simulink model "Arranque_exp"  (R2018b)
settings: Solver=VariableStepAuto  StartTime=0.0  StopTime=20  MaxStep=1e-4  RelTol=1e-3
values from neighbouring files (symbols this model uses):
  ia = a(:,2)-mean(a(:,2))    [carga_exp.m]
  ia1 = b(:,2)-mean(b(:,2))    [carga_exp.m]
  ib = a(:,4)-mean(a(:,4))    [carga_exp.m]
  ib1 = b(:,4)-mean(b(:,4))    [carga_exp.m]
  ic = a(:,3)-mean(a(:,3))    [carga_exp.m]
  ic1 = b(:,3)-mean(b(:,3))    [carga_exp.m]
  t1 = b(:,1)    [carga_exp.m]
  va = a(:,5)-mean(a(:,5))    [carga_exp.m]
  va1 = b(:,5)-mean(b(:,5))    [carga_exp.m]
  vb = a(:,7)-mean(a(:,7))    [carga_exp.m]
  vb1 = b(:,7)-mean(b(:,7))    [carga_exp.m]
  vc = a(:,6)-mean(a(:,6))    [carga_exp.m]
  vc1 = b(:,6)-mean(b(:,6))    [carga_exp.m]
libraries: powerlib_meascontrol x8
settings Model: Creator=Guille2  LastModifiedBy=grbos
settings SFSimCC: SimUseLocalCustomCode=off
settings RTWCC: RTWUseLocalCustomCode=off

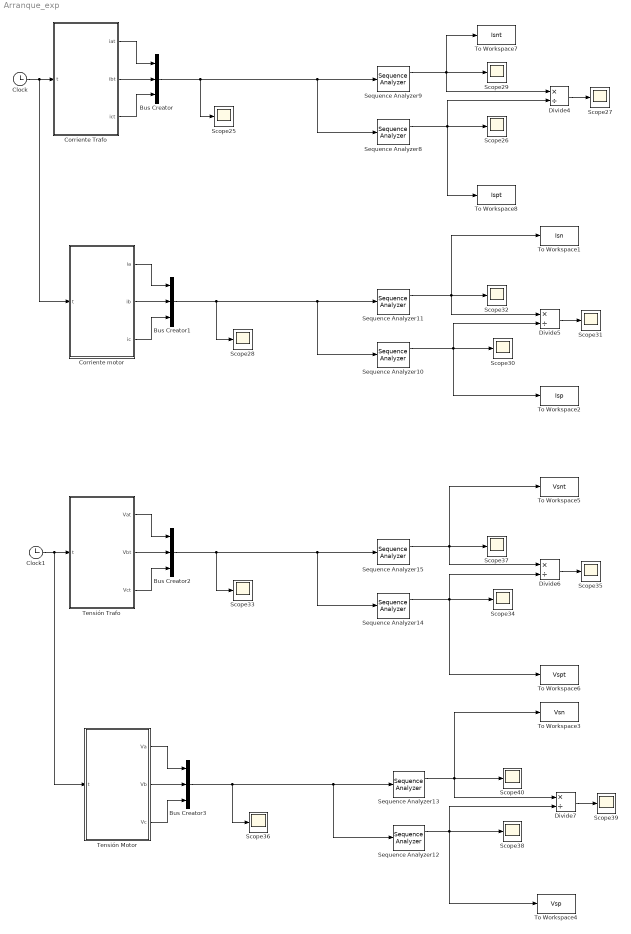
== system Arranque_exp ==
  Bus Creator{,1..3} (4 alike) : BusCreator  Inputs=3
  Clock : Clock
      settings: Decimation=20
  Clock1 : Clock
      settings: Decimation=20
  Corriente Trafo : Subsystem
  Corriente motor : Subsystem
  Divide{4..7} (4 alike) : Product  Inputs=*/
  Scope{25..40} (16 alike) : Scope
  Sequence Analyzer{8,10,12,14} (4 alike) : powerlib_meascontrol/Measurements/Sequence Analyzer  Freq=50  n=1  seq=Positive  InInit=[1, 0]  Ts=0
      settings: SourceProductName=Simscape Electrical  SourceProductBaseCode=PS
  Sequence Analyzer{9,11,13,15} (4 alike) : powerlib_meascontrol/Measurements/Sequence Analyzer  Freq=50  n=1  seq=Negative  InInit=[1, 0]  Ts=0
      settings: SourceProductName=Simscape Electrical  SourceProductBaseCode=PS
  Tensión Motor : Subsystem
  Tensión Trafo : Subsystem
  To Workspace1 : ToWorkspace  VariableName=Isn  SaveFormat=Timeseries  SampleTime=0.001
  To Workspace2 : ToWorkspace  VariableName=Isp  SaveFormat=Timeseries  SampleTime=0.001
  To Workspace3 : ToWorkspace  VariableName=Vsn  SaveFormat=Timeseries  SampleTime=0.001
  To Workspace4 : ToWorkspace  VariableName=Vsp  SaveFormat=Timeseries  SampleTime=0.001
  To Workspace5 : ToWorkspace  VariableName=Vsnt  SaveFormat=Timeseries  SampleTime=0.001
  To Workspace6 : ToWorkspace  VariableName=Vspt  SaveFormat=Timeseries  SampleTime=0.001
  To Workspace7 : ToWorkspace  VariableName=Isnt  SaveFormat=Timeseries  SampleTime=0.001
  To Workspace8 : ToWorkspace  VariableName=Ispt  SaveFormat=Timeseries  SampleTime=0.001
  wires:
  Corriente Trafo/1(iat) -> Bus Creator/1
  Corriente Trafo/2(ibt) -> Bus Creator/2
  Corriente Trafo/3(ict) -> Bus Creator/3
  Bus Creator/1 -> Sequence Analyzer8/1, Sequence Analyzer9/1, Scope25/1
  Clock/1 -> Corriente motor/1(t), Corriente Trafo/1(t)
  Sequence Analyzer8/1 -> Divide4/2, Scope26/1, To Workspace8/1
  Sequence Analyzer9/1 -> Divide4/1, Scope29/1, To Workspace7/1
  Divide4/1 -> Scope27/1
  Divide5/1 -> Scope31/1
  Sequence Analyzer11/1 -> Divide5/1, Scope32/1, To Workspace1/1
  Sequence Analyzer10/1 -> Divide5/2, Scope30/1, To Workspace2/1
  Bus Creator1/1 -> Sequence Analyzer10/1, Sequence Analyzer11/1, Scope28/1
  Corriente motor/1(ia) -> Bus Creator1/1
  Corriente motor/2(ib) -> Bus Creator1/2
  Corriente motor/3(ic) -> Bus Creator1/3
  Clock1/1 -> Tensión Motor/1(t), Tensión Trafo/1(t)
  Tensión Motor/2(Vb) -> Bus Creator3/2
  Tensión Trafo/3(Vct) -> Bus Creator2/3
  Divide6/1 -> Scope35/1
  Divide7/1 -> Scope39/1
  Bus Creator3/1 -> Sequence Analyzer12/1, Sequence Analyzer13/1, Scope36/1
  Tensión Trafo/2(Vbt) -> Bus Creator2/2
  Sequence Analyzer13/1 -> Divide7/1, Scope40/1, To Workspace3/1
  Tensión Trafo/1(Vat) -> Bus Creator2/1
  Sequence Analyzer12/1 -> Divide7/2, Scope38/1, To Workspace4/1
  Sequence Analyzer14/1 -> To Workspace6/1, Divide6/2, Scope34/1
  Tensión Motor/1(Va) -> Bus Creator3/1
  Bus Creator2/1 -> Sequence Analyzer14/1, Sequence Analyzer15/1, Scope33/1
  Tensión Motor/3(Vc) -> Bus Creator3/3
  Sequence Analyzer15/1 -> Divide6/1, Scope37/1, To Workspace5/1

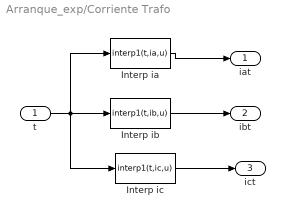
== system Arranque_exp/Corriente Trafo ==
  t : Inport
  Interp ia : MATLABFcn  MATLABFcn=interp1(t,ia,u)  OutputDimensions=1  OutputSignalType=real  Output1D=off
  Interp ib : MATLABFcn  MATLABFcn=interp1(t,ib,u)  OutputDimensions=1  OutputSignalType=real  Output1D=off
  Interp ic : MATLABFcn  MATLABFcn=interp1(t,ic,u)  OutputDimensions=1  Output1D=off
  iat : Outport
  ibt : Outport  Port=2
  ict : Outport  Port=3
  wires:
  Interp ia/1 -> iat/1
  Interp ib/1 -> ibt/1
  t/1 -> Interp ia/1, Interp ib/1, Interp ic/1
  Interp ic/1 -> ict/1

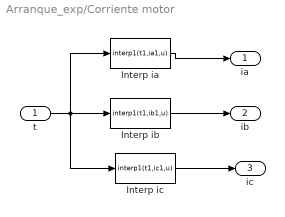
== system Arranque_exp/Corriente motor ==
  t : Inport
  Interp ia : MATLABFcn  MATLABFcn=interp1(t1,ia1,u)  OutputDimensions=1  OutputSignalType=real  Output1D=off
  Interp ib : MATLABFcn  MATLABFcn=interp1(t1,ib1,u)  OutputDimensions=1  OutputSignalType=real  Output1D=off
  Interp ic : MATLABFcn  MATLABFcn=interp1(t1,ic1,u)  OutputDimensions=1  Output1D=off
  ia : Outport
  ib : Outport  Port=2
  ic : Outport  Port=3
  wires:
  Interp ia/1 -> ia/1
  Interp ib/1 -> ib/1
  t/1 -> Interp ia/1, Interp ib/1, Interp ic/1
  Interp ic/1 -> ic/1

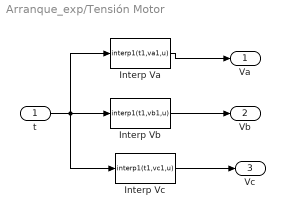
== system Arranque_exp/Tensión Motor ==
  t : Inport
  Interp Va : MATLABFcn  MATLABFcn=interp1(t1,va1,u)  OutputDimensions=1  OutputSignalType=real  Output1D=off
  Interp Vb : MATLABFcn  MATLABFcn=interp1(t1,vb1,u)  OutputDimensions=1  OutputSignalType=real  Output1D=off
  Interp Vc : MATLABFcn  MATLABFcn=interp1(t1,vc1,u)  OutputDimensions=1  Output1D=off
  Va : Outport
  Vb : Outport  Port=2
  Vc : Outport  Port=3
  wires:
  Interp Va/1 -> Va/1
  Interp Vb/1 -> Vb/1
  t/1 -> Interp Va/1, Interp Vb/1, Interp Vc/1
  Interp Vc/1 -> Vc/1

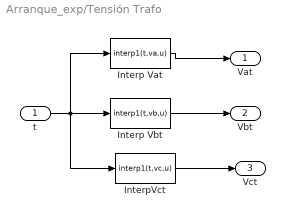
== system Arranque_exp/Tensión Trafo ==
  t : Inport
  Interp Vat : MATLABFcn  MATLABFcn=interp1(t,va,u)  OutputDimensions=1  OutputSignalType=real  Output1D=off
  Interp Vbt : MATLABFcn  MATLABFcn=interp1(t,vb,u)  OutputDimensions=1  OutputSignalType=real  Output1D=off
  InterpVct : MATLABFcn  MATLABFcn=interp1(t,vc,u)  OutputDimensions=1  Output1D=off
  Vat : Outport
  Vbt : Outport  Port=2
  Vct : Outport  Port=3
  wires:
  Interp Vat/1 -> Vat/1
  Interp Vbt/1 -> Vbt/1
  t/1 -> Interp Vat/1, Interp Vbt/1, InterpVct/1
  InterpVct/1 -> Vct/1
